simulink model "mbd3"  (R2021a)
settings: Solver=VariableStepAuto  StartTime=0.0  StopTime=10.0  RelTol=1e-3
settings Model: Creator=Shereen  LastModifiedBy=Shereen
settings HardwareCC: TargetBitPerPointer=64  TargetBitPerSizeT=64  TargetBitPerPtrDiffT=64  TargetLongLongMode=on  TargetIntDivRoundTo=Zero  TargetEndianess=LittleEndian  TargetWordSize=64  TargetHWDeviceType=MATLAB Host  ProdEqTarget=off
settings RTWCC: Description=Rapid Simulation Target  SystemTargetFile=rsim.tlc  TemplateMakefile=rsim_default_tmf
settings RSimTargetCC: TargetLangStandard=C99 (ISO)

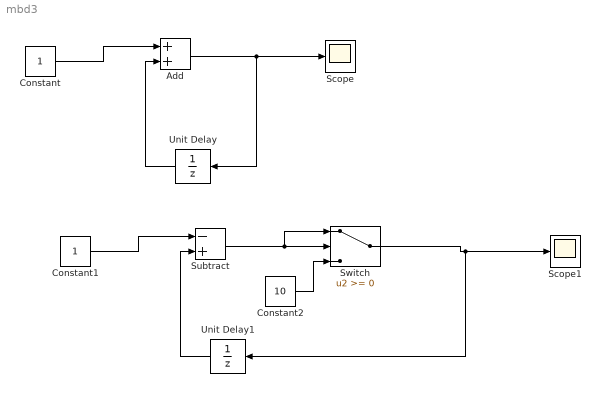
== system mbd3 ==
  Add : Sum
  Constant : Constant
  Constant1 : Constant
  Constant2 : Constant  Value=10
  Scope : Scope
  Scope1 : Scope
  Subtract : Sum  Inputs=-+
  Switch : Switch
  Unit Delay : UnitDelay  SampleTime=-1  HasFrameUpgradeWarning=on
  Unit Delay1 : UnitDelay  SampleTime=-1  HasFrameUpgradeWarning=on
  wires:
  Constant/1 -> Add/1
  Add/1 -> Scope/1, Unit Delay/1
  Unit Delay/1 -> Add/2
  Unit Delay1/1 -> Subtract/2
  Constant1/1 -> Subtract/1
  Subtract/1 -> Switch/1, Switch/2
  Constant2/1 -> Switch/3
  Switch/1 -> Unit Delay1/1, Scope1/1
